simulink model "v2_sim"  (R2023b)
settings: Solver=VariableStepAuto  StartTime=0.0  StopTime=30
values from neighbouring files (symbols this model uses):
  alpha = double(sol.alpha)    [WP4.m]
  beta = double(sol.beta)    [WP4.m]
libraries: simulink x1
settings Model: Creator=kiraa  LastModifiedBy=kiraa

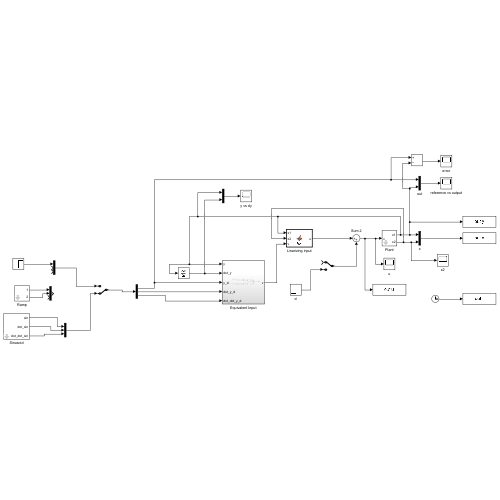
[thumbnail: Simulink's stored preview of the top-level diagram]
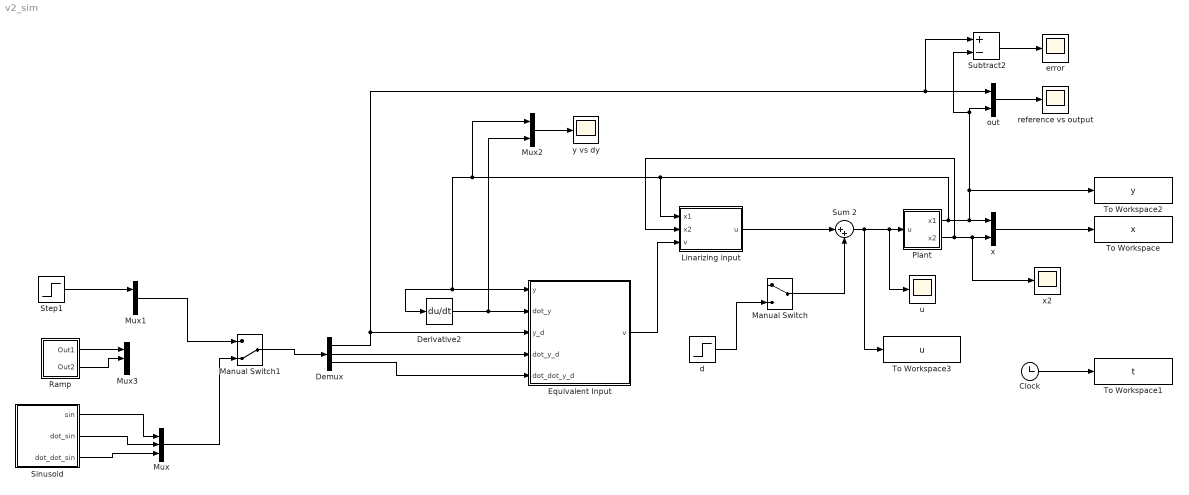
== system v2_sim ==
  Clock : Clock
  Demux : Demux  Outputs=3
  Derivative2 : Derivative
  Equivalent Input : Subsystem
  Linarizing input : MATLAB Function  TreatAsAtomicUnit=on
  Manual Switch : ManualSwitch
  Manual Switch1 : ManualSwitch  CurrentSetting=0
  Mux : Mux  Inputs=3
  Mux1 : Mux  Inputs=3
  Mux2 : Mux  Inputs=2
  Mux3 : Mux  Inputs=3
  Plant : Subsystem  mask{x1_0=0.001, x2_0=0.01}
      mask prompts: x1_0 "x1(0) [g/l]"; x2_0 "x2(0) [min^-1]"
  Ramp : Subsystem  mask{s=0.05}
      mask prompts: s "Slope"
  Sinusoid : Subsystem  mask{A=0.02, w=0.5, phi=0, b=0.0451}
      mask prompts: A "Amplitude"; w "Frequency [rad/s]"; phi "Phase"; b "Bias"
  Step1 : Step  Time=0  After=0.0451  SampleTime=0
  Subtract2 : Sum  Inputs=+-
  Sum 2 : Sum  Inputs=|++
  To Workspace : ToWorkspace  VariableName=x  SampleTime=-1
  To Workspace1 : ToWorkspace  VariableName=t  SaveFormat=Timeseries  SampleTime=-1
  To Workspace2 : ToWorkspace  VariableName=y  SampleTime=-1
  To Workspace3 : ToWorkspace  VariableName=u  SampleTime=-1
  d : Step  Time=0.5  After=20000  SampleTime=0
  error : Scope
  out : Mux  Inputs=2
  reference vs output : Scope
  u : Scope
  x : Mux  Inputs=2
  x2 : Scope
  y vs dy : Scope
  wires:
  Clock/1 -> To Workspace1/1
  Demux/1 -> Subtract2/1, out/1, Equivalent Input/3(y_d)
  x/1 -> To Workspace/1
  out/1 -> reference vs output/1
  Plant/1(x1) -> Derivative2/1, Equivalent Input/1(y), Mux2/1, Linarizing input/1(x1), To Workspace2/1, Subtract2/2, out/2, x/1
  Plant/2(x2) -> Linarizing input/2(x2), x2/1, x/2
  Sum 2/1 -> To Workspace3/1, Plant/1(u), u/1
  d/1 -> Manual Switch/2
  Manual Switch/1 -> Sum 2/2
  Derivative2/1 -> Equivalent Input/2(dot_y), Mux2/2
  Linarizing input/1(u) -> Sum 2/1
  Manual Switch1/1 -> Demux/1
  Mux/1 -> Manual Switch1/2
  Mux2/1 -> y vs dy/1
  Sinusoid/1(sin) -> Mux/1
  Sinusoid/2(dot_sin) -> Mux/2
  Sinusoid/3(dot_dot_sin) -> Mux/3
  Subtract2/1 -> error/1
  Step1/1 -> Mux1/1
  Ramp/1(Out1) -> Mux3/1
  Ramp/2(Out2) -> Mux3/2
  Mux1/1 -> Manual Switch1/1
  Demux/2 -> Equivalent Input/4(dot_y_d)
  Demux/3 -> Equivalent Input/5(dot_dot_y_d)
  Equivalent Input/1(v) -> Linarizing input/3(v)

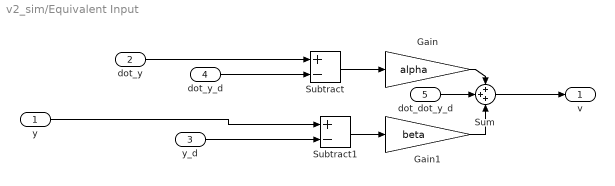
== system v2_sim/Equivalent Input ==
  y : Inport
  dot_y : Inport  Port=2
  y_d : Inport  Port=3
  dot_y_d : Inport  Port=4
  dot_dot_y_d : Inport  Port=5
  Gain : Gain  Gain=alpha
  Gain1 : Gain  Gain=beta
  Subtract : Sum  Inputs=+-
  Subtract1 : Sum  Inputs=+-
  Sum : Sum  Inputs=+++
  v : Outport
  wires:
  Gain/1 -> Sum/1
  Gain1/1 -> Sum/3
  Subtract/1 -> Gain/1
  Subtract1/1 -> Gain1/1
  dot_y_d/1 -> Subtract/2
  y/1 -> Subtract1/1
  dot_y/1 -> Subtract/1
  Sum/1 -> v/1
  y_d/1 -> Subtract1/2
  dot_dot_y_d/1 -> Sum/2

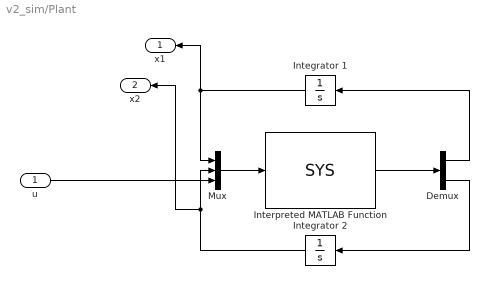
== system v2_sim/Plant ==
  u : Inport
  Demux : Demux  Outputs=2
  Integrator 1 : Integrator  InitialCondition=x1_0
  Integrator 2 : Integrator  InitialCondition=x2_0
  Interpreted MATLAB Function : MATLABFcn  MATLABFcn=SYS  OutputDimensions=2
  Mux : Mux  Inputs=3
  x1 : Outport
  x2 : Outport  Port=2
  wires:
  Integrator 1/1 -> x1/1, Mux/1
  Demux/1 -> Integrator 1/1
  Mux/1 -> Interpreted MATLAB Function/1
  Integrator 2/1 -> x2/1, Mux/2
  Interpreted MATLAB Function/1 -> Demux/1
  Demux/2 -> Integrator 2/1
  u/1 -> Mux/3

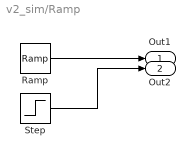
== system v2_sim/Ramp ==
  Ramp : simulink/Sources/Ramp  slope=s  start=0  InitialOutput=0
  Step : Step  Time=0  After=s  SampleTime=0
  Out1 : Outport
  Out2 : Outport  Port=2
  wires:
  Step/1 -> Out2/1
  Ramp/1 -> Out1/1

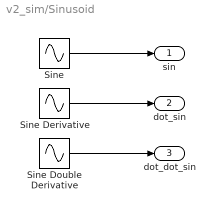
== system v2_sim/Sinusoid ==
  Sine : Sin  Amplitude=A  Bias=b  Frequency=w  Phase=phi  SampleTime=0
  Sine Derivative : Sin  Amplitude=-A*w  Frequency=w  Phase=phi-pi/2  SampleTime=0
  Sine Double Derivative : Sin  Amplitude=-A*w*w  Frequency=w  Phase=phi  SampleTime=0
  sin : Outport
  dot_sin : Outport  Port=2
  dot_dot_sin : Outport  Port=3
  wires:
  Sine Derivative/1 -> dot_sin/1
  Sine/1 -> sin/1
  Sine Double Derivative/1 -> dot_dot_sin/1

== matlab function v2_sim/Linarizing input ==
  data: x1 input; x2 input; v input; u output
function u = fcn(x1,x2,v)
    p1 = 0.0151; %tasso base di rimozione del glucosio dal sangue
    p2 = 0.0313; %tasso rimozione del glucosio dovuto all'insulina
    p3 = 0.0097;
    ge = 0.97;
    ie = 0.003;
    if x1 < 0.0000000001 %Messaggio di errore se lo stato x1 si annulla
        warning('The state x1 is approaching zero. This could led the system to explode.')
    end
    
    u = (1/(p3*x1))*((p1+x2)^2*x1-(p1+x2)*p1*ge+p2*x1*x2+p3*ie*x1-v);
    %fprintf("%.2f\n",u);
end
